simulink model "LinearInvPendSim"  (R2019a)
settings: Solver=ode45  StartTime=0.0  StopTime=3  RelTol=1e-3  EnableMultiTasking=on
values from neighbouring files (symbols this model uses):
  ref = -1    [LinearSim.m]
  sys = minreal(sys)    [LinearSim.m]
libraries: cstblocks x2, dspsrcs4 x1, simulink_extras x1
settings Model: Creator=FawaD KhaN  LastModifiedBy=FawadFarooq
settings DataIOCC: LimitDataPoints=on  SaveFormat=Array  ReturnWorkspaceOutputs=off
settings OptimizationCC: LifeSpan=inf
settings DebuggingCC: SFUnexpectedBacktrackingDiag=warning  SFNoUnconditionalDefaultTransitionDiag=warning  SFExecutionAtInitializationDiag=none  ArithmeticOperatorsInVariantConditions=warning
settings HardwareCC: ProdBitPerPointer=32  ProdBitPerSizeT=32  ProdBitPerPtrDiffT=32  ProdLargestAtomicFloat=None  ProdIntDivRoundTo=Undefined  ProdEndianess=Unspecified  ProdWordSize=32  ProdHWDeviceType=32-bit Generic
settings ModelReferenceCC: PropagateSignalLabelsOutOfModel=off
settings SFSimCC: SimUseLocalCustomCode=off
settings RTWCC: RTWUseLocalCustomCode=off
settings CodeAppCC: StateflowObjectComments=on
settings GRTTargetCC: TargetLangStandard=C89/C90 (ANSI)  GeneratePreprocessorConditionals=Disable all
settings ConfigComp: CovMetricSettings=dw  CovHtmlReporting=on  CovSaveCumulativeToWorkspaceVar=on  CovSaveSingleToWorkspaceVar=on  CovExternalEMLEnable=off

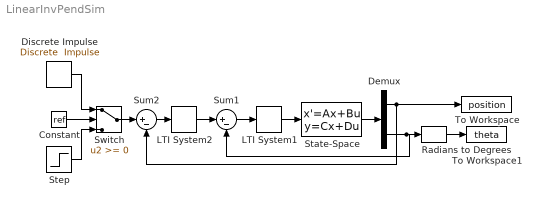
== system LinearInvPendSim ==
  Constant : Constant  Value=ref
  Demux : Demux  Outputs=2
  Discrete Impulse : dspsrcs4/Discrete  Impulse  Delay=0  SampleTime=0.1  FrameSample=1  OutputFrames=off  dataType=double  isSigned=on  wordLen=16  udDataType=sfix(16)  fracBitsMode=Best precision  numFracBits=15  OutDataTypeStr=double  LastOutDataTypeStr=double
  LTI System1 : cstblocks/LTI System  sys=Kth  IC=[]
  LTI System2 : cstblocks/LTI System  sys=Kx  IC=[]
  Radians to Degrees : simulink_extras/Transformations/Radians to Degrees
  State-Space : StateSpace  A=sys.A  B=sys.B  C=sys.C  D=sys.D  InitialCondition=0
  Step : Step  Time=0.1  SampleTime=0
  Sum1 : Sum  Inputs=|+-
  Sum2 : Sum  Inputs=|+-
  Switch : Switch
  To Workspace : ToWorkspace  VariableName=position  SaveFormat=Timeseries  SampleTime=-1
  To Workspace1 : ToWorkspace  VariableName=theta  SaveFormat=Timeseries  SampleTime=-1
  wires:
  Radians to Degrees/1 -> To Workspace1/1
  LTI System1/1 -> State-Space/1
  Sum1/1 -> LTI System1/1
  Demux/2 -> Radians to Degrees/1, Sum1/2
  Demux/1 -> To Workspace/1, Sum2/2
  State-Space/1 -> Demux/1
  Sum2/1 -> LTI System2/1
  LTI System2/1 -> Sum1/1
  Discrete Impulse/1 -> Switch/1
  Switch/1 -> Sum2/1
  Step/1 -> Switch/3
  Constant/1 -> Switch/2
